simulink library "Lib_Solve_OuterLoopIntegrator_TMATS"  (R2019b)
settings: Solver=ode45  StartTime=0.0  StopTime=10.0  RelTol=1e-3  EnableMultiTasking=on
Description:
  | Thomas Modules
settings Model: Creator=jwchapm2  LastModifiedBy=bhisma
settings DataIOCC: LimitDataPoints=on  SaveFormat=Array  ReturnWorkspaceOutputs=off
settings OptimizationCC: ExpressionDepthLimit=2147483647  LifeSpan=inf
settings DebuggingCC: UnderspecifiedInitializationDetection=Classic  MergeDetectMultiDrivingBlocksExec=none  SolverPrmCheckMsg=warning  StateNameClashWarn=warning  SFUnexpectedBacktrackingDiag=warning  SFNoUnconditionalDefaultTransitionDiag=warning  SFExecutionAtInitializationDiag=none  ArithmeticOperatorsInVariantConditions=warning
settings HardwareCC: ProdBitPerPointer=32  ProdBitPerSizeT=32  ProdBitPerPtrDiffT=32  ProdLargestAtomicFloat=None  ProdIntDivRoundTo=Undefined  ProdEndianess=Unspecified  ProdWordSize=32  ProdHWDeviceType=32-bit Generic
settings ModelReferenceCC: PropagateSignalLabelsOutOfModel=off
settings SFSimCC: SimUseLocalCustomCode=off  CustomCodeUndefinedFunction=UseInterfaceOnly
settings RTWCC: RTWUseLocalCustomCode=off
settings CodeAppCC: StateflowObjectComments=on
settings GRTTargetCC: TargetLangStandard=C89/C90 (ANSI)  GeneratePreprocessorConditionals=Disable all
settings ConfigComp: CovMetricSettings=dw  CovHtmlReporting=on  CovSaveCumulativeToWorkspaceVar=on  CovSaveSingleToWorkspaceVar=on  CovExternalEMLEnable=off

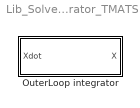
== system Lib_Solve_OuterLoopIntegrator_TMATS ==
  OuterLoop integrator : Subsystem  mask(T-MATS: OuterLoop Integrator Library Block){OL_IC_M=10000}
      mask prompts: OL_IC_M "OL_IC_M - Model Outer Loop Initial Conditions"
      mask help: Continuous-time integration of the input signal. To be used in the simulations outer, time based, loop.
      mask Help: web(which('Solver_TMATS_OLI.html'),'-helpbrowser')

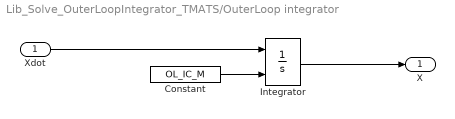
== system Lib_Solve_OuterLoopIntegrator_TMATS/OuterLoop integrator ==
  Xdot : Inport
  Constant : Constant  Value=OL_IC_M
  Integrator : Integrator  InitialConditionSource=external
  X : Outport
  wires:
  Constant/1 -> Integrator/2
  Xdot/1 -> Integrator/1
  Integrator/1 -> X/1
